simulink model "OpenSeesPy_Simulink"  (R2021a)
settings: Solver=ode8  StartTime=0.0  StopTime=31.2  FixedStep=dtfast  RelTol=1e-3
PreLoadFcn:
  | initializeSimulation;
InitFcn:
  | clear('all');
  | initializeSimulation;
undefined symbols (not defined in the file): adaptive, Area, areaC, asiv, Be, Cl, coef, damperA, damperB, damperC, damperCanon, denfilter, DiscIntNeverNeededParam, dtsim, f, fir_coef, flowCanon, forceCanon, forgfact, frictionA, frictionB, frictionC, gasConstant, Gsnsr_DT, Gsnsr_FT, Kc, ke, kgap, khard, Kp, Kq, kv, learningrate, lengthCanon, massA, massB, massC, massCanon, maxDisplA, maxDisplB, maxDisplC, maxForceC, maxOilVolume, maxVelocA, maxVelocB, maxVelocC, minDisplA, minDisplB, minDisplC, minVelocA, minVelocB, minVelocC, n1siv, n2siv, Ngap, nsiv, numfilter, P_corr_i, precharge, pumpFlow ... (+25)
libraries: simulink x4, instrumentlib x2, dsparch4 x1, sldrtlib x1
(part 2 of 3)

== system OpenSeesPy_Simulink/MTS actuator/static channel #3/payload ==
  force : Inport
  Sum : Sum  Inputs=+----  InputSameDT=on  SaturateOnIntegerOverflow=on  OutDataTypeStr=Inherit: Same as first input
  damper : Gain  Gain=damperC*damperCanon  SaturateOnIntegerOverflow=on  OutDataTypeStr=Inherit: Same as input  ParamDataTypeStr=Inherit: Same as input
  div : Product  Inputs=*/  InputSameDT=on  SaturateOnIntegerOverflow=on  OutDataTypeStr=Inherit: Same as first input
  double integrator : Subsystem
  friction : Subsystem  mask{friction=frictionC*forceCanon, yieldDispl=yieldDisplC*lengthCanon, hysteresis=0}
      mask prompts: friction "Sliding friction"; yieldDispl "Equiv. yield displacement (in)"; hysteresis "Hysteresis constant"
  mass : Constant  Value=massC*massCanon
  static force : Constant  Value=staticForceC*forceCanon
  term1 : Terminator
  unit dly : UnitDelay  SampleTime=-1  HasFrameUpgradeWarning=on
  unit dly1 : UnitDelay  SampleTime=-1  HasFrameUpgradeWarning=on
  veloc units : Gain  Gain=1/velocCanon  SaturateOnIntegerOverflow=on  OutDataTypeStr=Inherit: Same as input  ParamDataTypeStr=Inherit: Same as input
  displ : Outport
  veloc : Outport  Port=2
  tag scope: ch7a=global
  wires:
  unit dly/1 -> [ch7a]
  [ch7b] -> Sum/3  "spring force"
  unit dly1/1 -> damper/1
  damper/1 -> Sum/4  "damper force"
  static force/1 -> Sum/5  "static force"
  double integrator/2(veloc) -> unit dly1/1, friction/1(veloc), veloc units/1
  double integrator/1(displ) -> unit dly/1, displ/1
  div/1 -> double integrator/1(accel)
  double integrator/3(acc) -> term1/1
  mass/1 -> div/2
  force/1 -> Sum/1  "total force"
  Sum/1 -> div/1  "inertial force"
  veloc units/1 -> veloc/1
  friction/1(force) -> Sum/2  "friction force"

== system OpenSeesPy_Simulink/MTS actuator/static channel #4/actuator//valve model ==
  note: Parameter vector:
      | 1:   oil bulk modulus (force/displ^2)
      | 2:   servovalve delay (sec)
      | 3:   servovalve overlap
      | 4:   rated pressure (force/displ^2)
      | 5:   rated flow at rated pressure (displ^3/sec)
      | 6:   nominal flow at rated pressure (displ^3/sec)
      | 7:   actuator piston area 1 (displ^2)
      | 8:   actuator piston area 2 (displ^2)
      | 9:   actuator usable stroke 1 (displ)
      | 10: actuator usable stroke 2 (displ)
      | 11: actuator end cushion length 1 (displ)
      | 12: actuator end cushion length 2 (displ)
      | 13: actuator parasitic damping factor
      | 14: cross-chamber leakage factor (flow/press)
      | 15: ratio port openings according to area
      | 16: sample period (sec)
      |
      | Conversion factors used for converting
      | signals from external (user) to internal
      | (canonical) units:
      |
      | 17: displacement
      | 18: velocity
      | 19: force
      | 20: pressure
      | 21: flow
  note: Note: "1" and "2" denote actuator
      | cylinders on either side of the
      | actuator piston.  With positive
      | valve drive, oil is ported into
      | cylinder 1, resulting in positive
      | displacement.
  note: Auxiliary diagnostic output vector:
      | 1:   valve opening
      | 2:   C1 pressure
      | 3:   C2 pressure
      | 4:   delta pressure
      | 5:   force
      | 6:   velocity
      | 7:   C1 flow
      | 8:   C2 flow
      | 9:   total flow
      | 10: kinematic flow
      | 11: compressibility flow
      | 12: leakage flow
  cmd : Inport
  displ : Inport  Port=2
  veloc : Inport  Port=3
  spl press : Inport  Port=4
  rtn press : Inport  Port=5
  abs : Abs  SaturateOnIntegerOverflow=on
  actuator : S-Function  FunctionName=actuator  Parameters=actParamsC  SFunctionDeploymentMode=off  EnableBusSupport=off
  total flow sel : Selector  InputPortWidth=12  IndexOptions=Index vector (dialog)  Indices=9  OutputSizes=1
  force : Outport
  flow : Outport  Port=2
  wires:
  veloc/1 -> actuator/3
  displ/1 -> actuator/2
  actuator/1 -> force/1
  cmd/1 -> actuator/1
  rtn press/1 -> actuator/5
  spl press/1 -> actuator/4
  total flow sel/1 -> abs/1
  actuator/2 -> total flow sel/1
  abs/1 -> flow/1

== system OpenSeesPy_Simulink/MTS actuator/static channel #4/payload ==
  force : Inport
  Sum : Sum  Inputs=+----  InputSameDT=on  SaturateOnIntegerOverflow=on  OutDataTypeStr=Inherit: Same as first input
  damper : Gain  Gain=damperC*damperCanon  SaturateOnIntegerOverflow=on  OutDataTypeStr=Inherit: Same as input  ParamDataTypeStr=Inherit: Same as input
  div : Product  Inputs=*/  InputSameDT=on  SaturateOnIntegerOverflow=on  OutDataTypeStr=Inherit: Same as first input
  double integrator : Subsystem
  friction : Subsystem  mask{friction=frictionC*forceCanon, yieldDispl=yieldDisplC*lengthCanon, hysteresis=0}
      mask prompts: friction "Sliding friction"; yieldDispl "Equiv. yield displacement (in)"; hysteresis "Hysteresis constant"
  mass : Constant  Value=massC*massCanon
  static force : Constant  Value=staticForceC*forceCanon
  term1 : Terminator
  unit dly : UnitDelay  SampleTime=-1  HasFrameUpgradeWarning=on
  unit dly1 : UnitDelay  SampleTime=-1  HasFrameUpgradeWarning=on
  veloc units : Gain  Gain=1/velocCanon  SaturateOnIntegerOverflow=on  OutDataTypeStr=Inherit: Same as input  ParamDataTypeStr=Inherit: Same as input
  displ : Outport
  veloc : Outport  Port=2
  tag scope: ch8a=global
  wires:
  unit dly/1 -> [ch8a]
  [ch8b] -> Sum/3  "spring force"
  unit dly1/1 -> damper/1
  damper/1 -> Sum/4  "damper force"
  static force/1 -> Sum/5  "static force"
  double integrator/2(veloc) -> unit dly1/1, friction/1(veloc), veloc units/1
  double integrator/1(displ) -> unit dly/1, displ/1
  div/1 -> double integrator/1(accel)
  double integrator/3(acc) -> term1/1
  mass/1 -> div/2
  force/1 -> Sum/1  "total force"
  Sum/1 -> div/1  "inertial force"
  veloc units/1 -> veloc/1
  friction/1(force) -> Sum/2  "friction force"

== system OpenSeesPy_Simulink/Plant/Subsystem/Hardening-spring ==
  x : Inport
  Constant1 : Constant  Value=khard
  MATLAB Function : MATLAB Function  TreatAsAtomicUnit=on
  To Workspace : ToWorkspace  VariableName=Fhard  SaveFormat=Timeseries  SampleTime=-1
  Unit Delay : UnitDelay  SampleTime=-1  HasFrameUpgradeWarning=on
  Fhard : Outport  VectorParamsAs1DForOutWhenUnconnected=off
  wires:
  x/1 -> Unit Delay/1
  Constant1/1 -> MATLAB Function/2(khard)
  MATLAB Function/1(Fhard) -> Fhard/1, To Workspace/1
  Unit Delay/1 -> MATLAB Function/1(x)

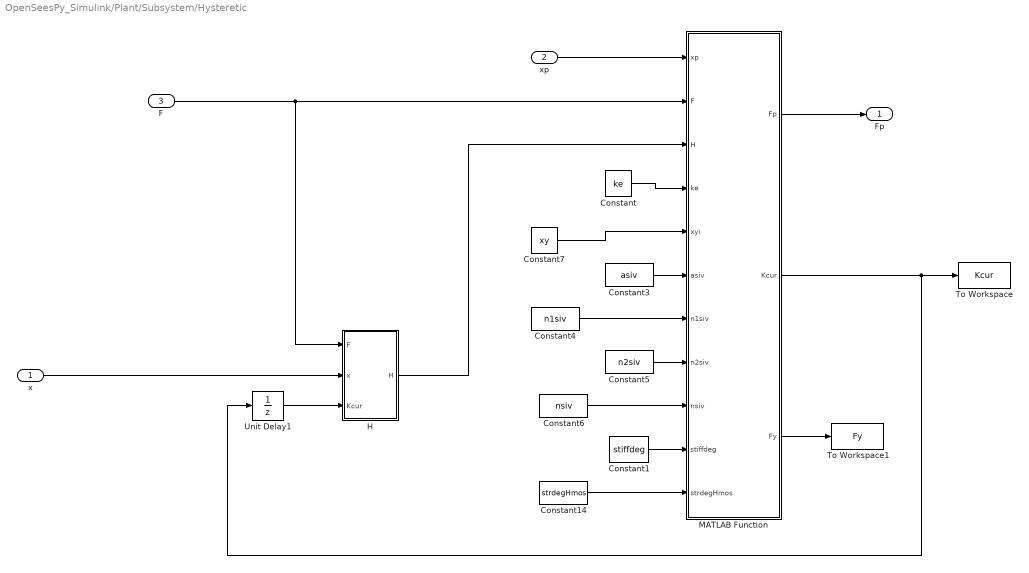
== system OpenSeesPy_Simulink/Plant/Subsystem/Hysteretic ==
  x : Inport
  xp : Inport  Port=2
  F : Inport  Port=3
  Constant : Constant  Value=ke
  Constant1 : Constant  Value=stiffdeg
  Constant14 : Constant  Value=strdegHmos
  Constant3 : Constant  Value=asiv
  Constant4 : Constant  Value=n1siv
  Constant5 : Constant  Value=n2siv
  Constant6 : Constant  Value=nsiv
  Constant7 : Constant  Value=xy
  H : Subsystem
  MATLAB Function : MATLAB Function  TreatAsAtomicUnit=on
  To Workspace : ToWorkspace  VariableName=Kcur  SaveFormat=Timeseries  SampleTime=-1
  To Workspace1 : ToWorkspace  VariableName=Fy  SaveFormat=Timeseries  SampleTime=-1
  Unit Delay1 : UnitDelay  InitialCondition=ke  SampleTime=-1  HasFrameUpgradeWarning=on
  Fp : Outport  VectorParamsAs1DForOutWhenUnconnected=off
  wires:
  MATLAB Function/1(Fp) -> Fp/1
  MATLAB Function/2(Kcur) -> To Workspace/1, Unit Delay1/1
  x/1 -> H/2(x)
  xp/1 -> MATLAB Function/1(xp)
  Constant/1 -> MATLAB Function/4(ke)
  Constant7/1 -> MATLAB Function/5(xyi)
  Constant1/1 -> MATLAB Function/10(stiffdeg)
  Constant3/1 -> MATLAB Function/6(asiv)
  Constant4/1 -> MATLAB Function/7(n1siv)
  Constant5/1 -> MATLAB Function/8(n2siv)
  Constant6/1 -> MATLAB Function/9(nsiv)
  H/1(H) -> MATLAB Function/3(H)
  Unit Delay1/1 -> H/3("Kcur ")
  F/1 -> MATLAB Function/2(F), H/1(F)
  MATLAB Function/3(Fy) -> To Workspace1/1
  Constant14/1 -> MATLAB Function/11(strdegHmos)

== system OpenSeesPy_Simulink/Plant/Subsystem/gapclosing ==
  x : Inport
  Constant : Constant  Value=ke
  Constant1 : Constant  Value=kgap
  Constant7 : Constant  Value=Ngap
  Constant8 : Constant  Value=xgap
  MATLAB Function : MATLAB Function  TreatAsAtomicUnit=on
  To Workspace : ToWorkspace  VariableName=Fgap  SaveFormat=Timeseries  SampleTime=-1
  Unit Delay : UnitDelay  SampleTime=-1  HasFrameUpgradeWarning=on
  Fgap : Outport  VectorParamsAs1DForOutWhenUnconnected=off
  wires:
  Constant7/1 -> MATLAB Function/4(Ngap)
  MATLAB Function/1(Fgap) -> To Workspace/1, Fgap/1
  Constant1/1 -> MATLAB Function/2(kgap)
  Constant8/1 -> MATLAB Function/5(xgap)
  Constant/1 -> MATLAB Function/3(ke)
  x/1 -> Unit Delay/1
  Unit Delay/1 -> MATLAB Function/1(x)

== system OpenSeesPy_Simulink/Wiener Implementation/Prediction_Adaptive_Fixed/Contador ==
  Add : Sum
  Constant1 : Constant
  Unit Delay : UnitDelay  SampleTime=-1  HasFrameUpgradeWarning=on
  Out1 : Outport
  wires:
  Unit Delay/1 -> Add/2
  Constant1/1 -> Add/1
  Add/1 -> Out1/1, Unit Delay/1

== system OpenSeesPy_Simulink/Wiener Implementation/Prediction_Adaptive_Fixed/If Action Subsystem ==
  Disp : Inport
  lambda : Inport  Port=2
  Disp_Pred : Inport  Port=3
  Action Port : ActionPort  ActionPortLabel=if(u1 <2)
  Add : Sum
  Buffer1 : Buffer  N=8  V=7  OutputFrames=off
  Constant1 : Constant
  Constant2 : Constant  Value=w_80
  Gain : Gain  Gain=1e-10
  Product : Product
  Product1 : Product  Inputs=3
  Sum : Sum  Inputs=|+-
  Sum1 : Sum  Inputs=|+-
  Unit Delay : UnitDelay  SampleTime=-1  HasFrameUpgradeWarning=on
  W_new : Outport
  wires:
  lambda/1 -> Product1/1, Gain/1
  Gain/1 -> Sum1/2
  Add/1 -> W_new/1
  Constant2/1 -> Product/1
  Buffer1/1 -> Product1/2
  Product1/1 -> Add/2
  Product/1 -> Add/1
  Disp/1 -> Buffer1/1, Sum/1
  Sum1/1 -> Product/2
  Sum/1 -> Product1/3
  Unit Delay/1 -> Sum/2
  Constant1/1 -> Sum1/1
  Disp_Pred/1 -> Unit Delay/1

== system OpenSeesPy_Simulink/Wiener Implementation/Prediction_Adaptive_Fixed/If Action Subsystem1 ==
  Disp : Inport
  W_prev : Inport  Port=2
  lambda : Inport  Port=3
  Disp_Pred : Inport  Port=4
  Action Port : ActionPort  ActionPortLabel=else
  Add : Sum
  Buffer1 : Buffer  N=8  V=7  OutputFrames=off
  Constant1 : Constant
  Gain : Gain  Gain=1e-10
  Product : Product
  Product1 : Product  Inputs=3
  Sum : Sum  Inputs=|+-
  Sum1 : Sum  Inputs=|+-
  Unit Delay : UnitDelay  SampleTime=-1  HasFrameUpgradeWarning=on
  W_new : Outport
  wires:
  lambda/1 -> Product1/1, Gain/1
  Gain/1 -> Sum1/2
  Add/1 -> W_new/1
  W_prev/1 -> Product/1
  Buffer1/1 -> Product1/2
  Product1/1 -> Add/2
  Product/1 -> Add/1
  Disp/1 -> Buffer1/1, Sum/1
  Sum1/1 -> Product/2
  Sum/1 -> Product1/3
  Unit Delay/1 -> Sum/2
  Constant1/1 -> Sum1/1
  Disp_Pred/1 -> Unit Delay/1

== system OpenSeesPy_Simulink/Wiener Implementation/Test3/Subsystem ==
  Constant1 : Constant
  Constant3 : Constant  Value=2
  Constant5 : Constant  Value=3
  Constant6 : Constant  Value=0
  Constant7 : Constant  Value=x02
  Math Function{,1..3} (4 alike) : Math  Operator=pow  SaturateOnIntegerOverflow=on
  Matrix Concatenate : Concatenate  NumInputs=4  Mode=Multidimensional array  ConcatenateDimension=2
  a : Outport
  wires:
  Constant6/1 -> Math Function/2
  Constant1/1 -> Math Function1/2
  Constant3/1 -> Math Function2/2
  Constant5/1 -> Math Function3/2
  Math Function/1 -> Matrix Concatenate/1
  Math Function1/1 -> Matrix Concatenate/2
  Math Function2/1 -> Matrix Concatenate/3
  Math Function3/1 -> Matrix Concatenate/4
  Matrix Concatenate/1 -> a/1  "a"
  Constant7/1 -> Math Function3/1, Math Function2/1, Math Function1/1, Math Function/1

== system OpenSeesPy_Simulink/MTS actuator/dynamic long channel #1/payload/double integrator ==
  accel : Inport
  displ gen : DiscreteIntegrator  IntegratorMethod=Integration: Backward Euler  SampleTime=1/4000  LimitOutput=on  UpperSaturationLimit=maxDisplB*coef  LowerSaturationLimit=minDisplB*coef  ShowSaturationPort=on  ICPrevOutput=DiscIntNeverNeededParam  ICPrevScaledInput=DiscIntNeverNeededParam
  veloc gen : Subsystem  mask{maxVeloc=maxVelocB*velocCanon*coef, minVeloc=minVelocB*velocCanon*coef, maxDispl=maxDisplB*coef, minDispl=minDisplB*coef}
      mask prompts: maxVeloc "Max velocity"; minVeloc "Min velocity"; maxDispl "Max displacement"; minDispl "Min displacement"
  displ : Outport
  veloc : Outport  Port=2
  acc : Outport  Port=3
  wires:
  accel/1 -> acc/1, veloc gen/1(accel)
  veloc gen/1(veloc) -> veloc/1, displ gen/1
  displ gen/1 -> veloc gen/2(displ), displ/1
  displ gen/2 -> veloc gen/3(reset)

== system OpenSeesPy_Simulink/MTS actuator/dynamic long channel #1/payload/friction ==
  veloc : Inport
  1-beta : Gain  Gain=1-hysteresis  SaturateOnIntegerOverflow=on  OutDataTypeStr=Inherit: Same as input  ParamDataTypeStr=Inherit: Same as input
  Sign : Signum
  Sum : Sum  Inputs=|++  SaturateOnIntegerOverflow=on
  Sum1 : Sum  Inputs=|+-  SaturateOnIntegerOverflow=on
  beta : Constant  Value=hysteresis
  integrator : DiscreteIntegrator  SampleTime=-1  LimitOutput=on  UpperSaturationLimit=1  LowerSaturationLimit=-1  ICPrevOutput=DiscIntNeverNeededParam  ICPrevScaledInput=DiscIntNeverNeededParam
  one : Constant
  prod1 : Product  InputSameDT=on  SaturateOnIntegerOverflow=on  OutDataTypeStr=Inherit: Same as first input
  prod2 : Product  InputSameDT=on  SaturateOnIntegerOverflow=on  OutDataTypeStr=Inherit: Same as first input
  prod3 : Product  Inputs=3  InputSameDT=on  SaturateOnIntegerOverflow=on  OutDataTypeStr=Inherit: Same as first input
  prod4 : Product  InputSameDT=on  SaturateOnIntegerOverflow=on  OutDataTypeStr=Inherit: Same as first input
  sliding friction : Constant  Value=friction
  y inv : Gain  Gain=1/max(eps, yieldDispl)  SaturateOnIntegerOverflow=on  OutDataTypeStr=Inherit: Same as input  ParamDataTypeStr=Inherit: Same as input
  force : Outport
  wires:
  integrator/1 -> prod3/2, prod3/1, prod4/1, prod1/2  "zee"
  y inv/1 -> integrator/1
  prod2/1 -> y inv/1
  Sum1/1 -> prod2/1
  prod3/1 -> Sum1/2
  one/1 -> Sum1/1
  Sum/1 -> prod3/3
  beta/1 -> Sum/1
  1-beta/1 -> Sum/2
  Sign/1 -> 1-beta/1
  prod4/1 -> Sign/1
  veloc/1 -> prod2/2, prod4/2
  prod1/1 -> force/1
  sliding friction/1 -> prod1/1

== system OpenSeesPy_Simulink/MTS actuator/dynamic long channel #2/payload/double integrator ==
  accel : Inport
  displ gen : DiscreteIntegrator  IntegratorMethod=Integration: Backward Euler  SampleTime=-1  LimitOutput=on  UpperSaturationLimit=maxDisplB  LowerSaturationLimit=minDisplB  ShowSaturationPort=on  ICPrevOutput=DiscIntNeverNeededParam  ICPrevScaledInput=DiscIntNeverNeededParam
  veloc gen : Subsystem  mask{maxVeloc=maxVelocB*velocCanon, minVeloc=minVelocB*velocCanon, maxDispl=maxDisplB, minDispl=minDisplB}
      mask prompts: maxVeloc "Max velocity"; minVeloc "Min velocity"; maxDispl "Max displacement"; minDispl "Min displacement"
  displ : Outport
  veloc : Outport  Port=2
  acc : Outport  Port=3
  wires:
  accel/1 -> acc/1, veloc gen/1(accel)
  veloc gen/1(veloc) -> veloc/1, displ gen/1
  displ gen/1 -> veloc gen/2(displ), displ/1
  displ gen/2 -> veloc gen/3(reset)

== system OpenSeesPy_Simulink/MTS actuator/dynamic long channel #2/payload/friction ==
  veloc : Inport
  1-beta : Gain  Gain=1-hysteresis  SaturateOnIntegerOverflow=on  OutDataTypeStr=Inherit: Same as input  ParamDataTypeStr=Inherit: Same as input
  Sign : Signum
  Sum : Sum  Inputs=|++  SaturateOnIntegerOverflow=on
  Sum1 : Sum  Inputs=|+-  SaturateOnIntegerOverflow=on
  beta : Constant  Value=hysteresis
  integrator : DiscreteIntegrator  SampleTime=-1  LimitOutput=on  UpperSaturationLimit=1  LowerSaturationLimit=-1  ICPrevOutput=DiscIntNeverNeededParam  ICPrevScaledInput=DiscIntNeverNeededParam
  one : Constant
  prod1 : Product  InputSameDT=on  SaturateOnIntegerOverflow=on  OutDataTypeStr=Inherit: Same as first input
  prod2 : Product  InputSameDT=on  SaturateOnIntegerOverflow=on  OutDataTypeStr=Inherit: Same as first input
  prod3 : Product  Inputs=3  InputSameDT=on  SaturateOnIntegerOverflow=on  OutDataTypeStr=Inherit: Same as first input
  prod4 : Product  InputSameDT=on  SaturateOnIntegerOverflow=on  OutDataTypeStr=Inherit: Same as first input
  sliding friction : Constant  Value=friction
  y inv : Gain  Gain=1/max(eps, yieldDispl)  SaturateOnIntegerOverflow=on  OutDataTypeStr=Inherit: Same as input  ParamDataTypeStr=Inherit: Same as input
  force : Outport
  wires:
  integrator/1 -> prod3/2, prod3/1, prod4/1, prod1/2  "zee"
  y inv/1 -> integrator/1
  prod2/1 -> y inv/1
  Sum1/1 -> prod2/1
  prod3/1 -> Sum1/2
  one/1 -> Sum1/1
  Sum/1 -> prod3/3
  beta/1 -> Sum/1
  1-beta/1 -> Sum/2
  Sign/1 -> 1-beta/1
  prod4/1 -> Sign/1
  veloc/1 -> prod2/2, prod4/2
  prod1/1 -> force/1
  sliding friction/1 -> prod1/1

== system OpenSeesPy_Simulink/MTS actuator/dynamic short channel #1/payload/double integrator ==
  accel : Inport
  displ gen : DiscreteIntegrator  IntegratorMethod=Integration: Backward Euler  SampleTime=1/1024  LimitOutput=on  UpperSaturationLimit=maxDisplA  LowerSaturationLimit=minDisplA  ShowSaturationPort=on  ICPrevOutput=DiscIntNeverNeededParam  ICPrevScaledInput=DiscIntNeverNeededParam
  veloc gen : Subsystem  mask{maxVeloc=maxVelocA*velocCanon, minVeloc=minVelocA*velocCanon, maxDispl=maxDisplA, minDispl=minDisplA}
      mask prompts: maxVeloc "Max velocity"; minVeloc "Min velocity"; maxDispl "Max displacement"; minDispl "Min displacement"
  displ : Outport
  veloc : Outport  Port=2
  acc : Outport  Port=3
  wires:
  accel/1 -> acc/1, veloc gen/1(accel)
  veloc gen/1(veloc) -> veloc/1, displ gen/1
  displ gen/1 -> veloc gen/2(displ), displ/1
  displ gen/2 -> veloc gen/3(reset)

== system OpenSeesPy_Simulink/MTS actuator/dynamic short channel #1/payload/friction ==
  veloc : Inport
  1-beta : Gain  Gain=1-hysteresis  SaturateOnIntegerOverflow=on  OutDataTypeStr=Inherit: Same as input  ParamDataTypeStr=Inherit: Same as input
  Sign : Signum
  Sum : Sum  Inputs=|++  SaturateOnIntegerOverflow=on
  Sum1 : Sum  Inputs=|+-  SaturateOnIntegerOverflow=on
  beta : Constant  Value=hysteresis
  integrator : DiscreteIntegrator  SampleTime=-1  LimitOutput=on  UpperSaturationLimit=1  LowerSaturationLimit=-1  ICPrevOutput=DiscIntNeverNeededParam  ICPrevScaledInput=DiscIntNeverNeededParam
  one : Constant
  prod1 : Product  InputSameDT=on  SaturateOnIntegerOverflow=on  OutDataTypeStr=Inherit: Same as first input
  prod2 : Product  InputSameDT=on  SaturateOnIntegerOverflow=on  OutDataTypeStr=Inherit: Same as first input
  prod3 : Product  Inputs=3  InputSameDT=on  SaturateOnIntegerOverflow=on  OutDataTypeStr=Inherit: Same as first input
  prod4 : Product  InputSameDT=on  SaturateOnIntegerOverflow=on  OutDataTypeStr=Inherit: Same as first input
  sliding friction : Constant  Value=friction
  y inv : Gain  Gain=1/max(eps, yieldDispl)  SaturateOnIntegerOverflow=on  OutDataTypeStr=Inherit: Same as input  ParamDataTypeStr=Inherit: Same as input
  force : Outport
  wires:
  integrator/1 -> prod3/2, prod3/1, prod4/1, prod1/2  "zee"
  y inv/1 -> integrator/1
  prod2/1 -> y inv/1
  Sum1/1 -> prod2/1
  prod3/1 -> Sum1/2
  one/1 -> Sum1/1
  Sum/1 -> prod3/3
  beta/1 -> Sum/1
  1-beta/1 -> Sum/2
  Sign/1 -> 1-beta/1
  prod4/1 -> Sign/1
  veloc/1 -> prod2/2, prod4/2
  prod1/1 -> force/1
  sliding friction/1 -> prod1/1

== system OpenSeesPy_Simulink/MTS actuator/dynamic short channel #2/payload/double integrator ==
  accel : Inport
  displ gen : DiscreteIntegrator  IntegratorMethod=Integration: Backward Euler  SampleTime=-1  LimitOutput=on  UpperSaturationLimit=maxDisplA  LowerSaturationLimit=minDisplA  ShowSaturationPort=on  ICPrevOutput=DiscIntNeverNeededParam  ICPrevScaledInput=DiscIntNeverNeededParam
  veloc gen : Subsystem  mask{maxVeloc=maxVelocA*velocCanon, minVeloc=minVelocA*velocCanon, maxDispl=maxDisplA, minDispl=minDisplA}
      mask prompts: maxVeloc "Max velocity"; minVeloc "Min velocity"; maxDispl "Max displacement"; minDispl "Min displacement"
  displ : Outport
  veloc : Outport  Port=2
  acc : Outport  Port=3
  wires:
  accel/1 -> acc/1, veloc gen/1(accel)
  veloc gen/1(veloc) -> veloc/1, displ gen/1
  displ gen/1 -> veloc gen/2(displ), displ/1
  displ gen/2 -> veloc gen/3(reset)

== system OpenSeesPy_Simulink/MTS actuator/dynamic short channel #2/payload/friction ==
  veloc : Inport
  1-beta : Gain  Gain=1-hysteresis  SaturateOnIntegerOverflow=on  OutDataTypeStr=Inherit: Same as input  ParamDataTypeStr=Inherit: Same as input
  Sign : Signum
  Sum : Sum  Inputs=|++  SaturateOnIntegerOverflow=on
  Sum1 : Sum  Inputs=|+-  SaturateOnIntegerOverflow=on
  beta : Constant  Value=hysteresis
  integrator : DiscreteIntegrator  SampleTime=-1  LimitOutput=on  UpperSaturationLimit=1  LowerSaturationLimit=-1  ICPrevOutput=DiscIntNeverNeededParam  ICPrevScaledInput=DiscIntNeverNeededParam
  one : Constant
  prod1 : Product  InputSameDT=on  SaturateOnIntegerOverflow=on  OutDataTypeStr=Inherit: Same as first input
  prod2 : Product  InputSameDT=on  SaturateOnIntegerOverflow=on  OutDataTypeStr=Inherit: Same as first input
  prod3 : Product  Inputs=3  InputSameDT=on  SaturateOnIntegerOverflow=on  OutDataTypeStr=Inherit: Same as first input
  prod4 : Product  InputSameDT=on  SaturateOnIntegerOverflow=on  OutDataTypeStr=Inherit: Same as first input
  sliding friction : Constant  Value=friction
  y inv : Gain  Gain=1/max(eps, yieldDispl)  SaturateOnIntegerOverflow=on  OutDataTypeStr=Inherit: Same as input  ParamDataTypeStr=Inherit: Same as input
  force : Outport
  wires:
  integrator/1 -> prod3/2, prod3/1, prod4/1, prod1/2  "zee"
  y inv/1 -> integrator/1
  prod2/1 -> y inv/1
  Sum1/1 -> prod2/1
  prod3/1 -> Sum1/2
  one/1 -> Sum1/1
  Sum/1 -> prod3/3
  beta/1 -> Sum/1
  1-beta/1 -> Sum/2
  Sign/1 -> 1-beta/1
  prod4/1 -> Sign/1
  veloc/1 -> prod2/2, prod4/2
  prod1/1 -> force/1
  sliding friction/1 -> prod1/1

== system OpenSeesPy_Simulink/MTS actuator/static channel #1/payload/double integrator ==
  accel : Inport
  displ gen : DiscreteIntegrator  IntegratorMethod=Integration: Backward Euler  SampleTime=-1  LimitOutput=on  UpperSaturationLimit=maxDisplC  LowerSaturationLimit=minDisplC  ShowSaturationPort=on  ICPrevOutput=DiscIntNeverNeededParam  ICPrevScaledInput=DiscIntNeverNeededParam
  veloc gen : Subsystem  mask{maxVeloc=maxVelocC*velocCanon, minVeloc=minVelocC*velocCanon, maxDispl=maxDisplC, minDispl=minDisplC}
      mask prompts: maxVeloc "Max velocity"; minVeloc "Min velocity"; maxDispl "Max displacement"; minDispl "Min displacement"
  displ : Outport
  veloc : Outport  Port=2
  acc : Outport  Port=3
  wires:
  accel/1 -> acc/1, veloc gen/1(accel)
  veloc gen/1(veloc) -> veloc/1, displ gen/1
  displ gen/1 -> veloc gen/2(displ), displ/1
  displ gen/2 -> veloc gen/3(reset)

== system OpenSeesPy_Simulink/MTS actuator/static channel #1/payload/friction ==
  veloc : Inport
  1-beta : Gain  Gain=1-hysteresis  SaturateOnIntegerOverflow=on  OutDataTypeStr=Inherit: Same as input  ParamDataTypeStr=Inherit: Same as input
  Sign : Signum
  Sum : Sum  Inputs=|++  SaturateOnIntegerOverflow=on
  Sum1 : Sum  Inputs=|+-  SaturateOnIntegerOverflow=on
  beta : Constant  Value=hysteresis
  integrator : DiscreteIntegrator  SampleTime=-1  LimitOutput=on  UpperSaturationLimit=1  LowerSaturationLimit=-1  ICPrevOutput=DiscIntNeverNeededParam  ICPrevScaledInput=DiscIntNeverNeededParam
  one : Constant
  prod1 : Product  InputSameDT=on  SaturateOnIntegerOverflow=on  OutDataTypeStr=Inherit: Same as first input
  prod2 : Product  InputSameDT=on  SaturateOnIntegerOverflow=on  OutDataTypeStr=Inherit: Same as first input
  prod3 : Product  Inputs=3  InputSameDT=on  SaturateOnIntegerOverflow=on  OutDataTypeStr=Inherit: Same as first input
  prod4 : Product  InputSameDT=on  SaturateOnIntegerOverflow=on  OutDataTypeStr=Inherit: Same as first input
  sliding friction : Constant  Value=friction
  y inv : Gain  Gain=1/max(eps, yieldDispl)  SaturateOnIntegerOverflow=on  OutDataTypeStr=Inherit: Same as input  ParamDataTypeStr=Inherit: Same as input
  force : Outport
  wires:
  integrator/1 -> prod3/2, prod3/1, prod4/1, prod1/2  "zee"
  y inv/1 -> integrator/1
  prod2/1 -> y inv/1
  Sum1/1 -> prod2/1
  prod3/1 -> Sum1/2
  one/1 -> Sum1/1
  Sum/1 -> prod3/3
  beta/1 -> Sum/1
  1-beta/1 -> Sum/2
  Sign/1 -> 1-beta/1
  prod4/1 -> Sign/1
  veloc/1 -> prod2/2, prod4/2
  prod1/1 -> force/1
  sliding friction/1 -> prod1/1

== system OpenSeesPy_Simulink/MTS actuator/static channel #2/payload/double integrator ==
  accel : Inport
  displ gen : DiscreteIntegrator  IntegratorMethod=Integration: Backward Euler  SampleTime=-1  LimitOutput=on  UpperSaturationLimit=maxDisplC  LowerSaturationLimit=minDisplC  ShowSaturationPort=on  ICPrevOutput=DiscIntNeverNeededParam  ICPrevScaledInput=DiscIntNeverNeededParam
  veloc gen : Subsystem  mask{maxVeloc=maxVelocC*velocCanon, minVeloc=minVelocC*velocCanon, maxDispl=maxDisplC, minDispl=minDisplC}
      mask prompts: maxVeloc "Max velocity"; minVeloc "Min velocity"; maxDispl "Max displacement"; minDispl "Min displacement"
  displ : Outport
  veloc : Outport  Port=2
  acc : Outport  Port=3
  wires:
  accel/1 -> acc/1, veloc gen/1(accel)
  veloc gen/1(veloc) -> veloc/1, displ gen/1
  displ gen/1 -> veloc gen/2(displ), displ/1
  displ gen/2 -> veloc gen/3(reset)

== system OpenSeesPy_Simulink/MTS actuator/static channel #2/payload/friction ==
  veloc : Inport
  1-beta : Gain  Gain=1-hysteresis  SaturateOnIntegerOverflow=on  OutDataTypeStr=Inherit: Same as input  ParamDataTypeStr=Inherit: Same as input
  Sign : Signum
  Sum : Sum  Inputs=|++  SaturateOnIntegerOverflow=on
  Sum1 : Sum  Inputs=|+-  SaturateOnIntegerOverflow=on
  beta : Constant  Value=hysteresis
  integrator : DiscreteIntegrator  SampleTime=-1  LimitOutput=on  UpperSaturationLimit=1  LowerSaturationLimit=-1  ICPrevOutput=DiscIntNeverNeededParam  ICPrevScaledInput=DiscIntNeverNeededParam
  one : Constant
  prod1 : Product  InputSameDT=on  SaturateOnIntegerOverflow=on  OutDataTypeStr=Inherit: Same as first input
  prod2 : Product  InputSameDT=on  SaturateOnIntegerOverflow=on  OutDataTypeStr=Inherit: Same as first input
  prod3 : Product  Inputs=3  InputSameDT=on  SaturateOnIntegerOverflow=on  OutDataTypeStr=Inherit: Same as first input
  prod4 : Product  InputSameDT=on  SaturateOnIntegerOverflow=on  OutDataTypeStr=Inherit: Same as first input
  sliding friction : Constant  Value=friction
  y inv : Gain  Gain=1/max(eps, yieldDispl)  SaturateOnIntegerOverflow=on  OutDataTypeStr=Inherit: Same as input  ParamDataTypeStr=Inherit: Same as input
  force : Outport
  wires:
  integrator/1 -> prod3/2, prod3/1, prod4/1, prod1/2  "zee"
  y inv/1 -> integrator/1
  prod2/1 -> y inv/1
  Sum1/1 -> prod2/1
  prod3/1 -> Sum1/2
  one/1 -> Sum1/1
  Sum/1 -> prod3/3
  beta/1 -> Sum/1
  1-beta/1 -> Sum/2
  Sign/1 -> 1-beta/1
  prod4/1 -> Sign/1
  veloc/1 -> prod2/2, prod4/2
  prod1/1 -> force/1
  sliding friction/1 -> prod1/1

== system OpenSeesPy_Simulink/MTS actuator/static channel #3/payload/double integrator ==
  accel : Inport
  displ gen : DiscreteIntegrator  IntegratorMethod=Integration: Backward Euler  SampleTime=-1  LimitOutput=on  UpperSaturationLimit=maxDisplC  LowerSaturationLimit=minDisplC  ShowSaturationPort=on  ICPrevOutput=DiscIntNeverNeededParam  ICPrevScaledInput=DiscIntNeverNeededParam
  veloc gen : Subsystem  mask{maxVeloc=maxVelocC*velocCanon, minVeloc=minVelocC*velocCanon, maxDispl=maxDisplC, minDispl=minDisplC}
      mask prompts: maxVeloc "Max velocity"; minVeloc "Min velocity"; maxDispl "Max displacement"; minDispl "Min displacement"
  displ : Outport
  veloc : Outport  Port=2
  acc : Outport  Port=3
  wires:
  accel/1 -> acc/1, veloc gen/1(accel)
  veloc gen/1(veloc) -> veloc/1, displ gen/1
  displ gen/1 -> veloc gen/2(displ), displ/1
  displ gen/2 -> veloc gen/3(reset)

== system OpenSeesPy_Simulink/MTS actuator/static channel #3/payload/friction ==
  veloc : Inport
  1-beta : Gain  Gain=1-hysteresis  SaturateOnIntegerOverflow=on  OutDataTypeStr=Inherit: Same as input  ParamDataTypeStr=Inherit: Same as input
  Sign : Signum
  Sum : Sum  Inputs=|++  SaturateOnIntegerOverflow=on
  Sum1 : Sum  Inputs=|+-  SaturateOnIntegerOverflow=on
  beta : Constant  Value=hysteresis
  integrator : DiscreteIntegrator  SampleTime=-1  LimitOutput=on  UpperSaturationLimit=1  LowerSaturationLimit=-1  ICPrevOutput=DiscIntNeverNeededParam  ICPrevScaledInput=DiscIntNeverNeededParam
  one : Constant
  prod1 : Product  InputSameDT=on  SaturateOnIntegerOverflow=on  OutDataTypeStr=Inherit: Same as first input
  prod2 : Product  InputSameDT=on  SaturateOnIntegerOverflow=on  OutDataTypeStr=Inherit: Same as first input
  prod3 : Product  Inputs=3  InputSameDT=on  SaturateOnIntegerOverflow=on  OutDataTypeStr=Inherit: Same as first input
  prod4 : Product  InputSameDT=on  SaturateOnIntegerOverflow=on  OutDataTypeStr=Inherit: Same as first input
  sliding friction : Constant  Value=friction
  y inv : Gain  Gain=1/max(eps, yieldDispl)  SaturateOnIntegerOverflow=on  OutDataTypeStr=Inherit: Same as input  ParamDataTypeStr=Inherit: Same as input
  force : Outport
  wires:
  integrator/1 -> prod3/2, prod3/1, prod4/1, prod1/2  "zee"
  y inv/1 -> integrator/1
  prod2/1 -> y inv/1
  Sum1/1 -> prod2/1
  prod3/1 -> Sum1/2
  one/1 -> Sum1/1
  Sum/1 -> prod3/3
  beta/1 -> Sum/1
  1-beta/1 -> Sum/2
  Sign/1 -> 1-beta/1
  prod4/1 -> Sign/1
  veloc/1 -> prod2/2, prod4/2
  prod1/1 -> force/1
  sliding friction/1 -> prod1/1

== system OpenSeesPy_Simulink/MTS actuator/static channel #4/payload/double integrator ==
  accel : Inport
  displ gen : DiscreteIntegrator  IntegratorMethod=Integration: Backward Euler  SampleTime=-1  LimitOutput=on  UpperSaturationLimit=maxDisplC  LowerSaturationLimit=minDisplC  ShowSaturationPort=on  ICPrevOutput=DiscIntNeverNeededParam  ICPrevScaledInput=DiscIntNeverNeededParam
  veloc gen : Subsystem  mask{maxVeloc=maxVelocC*velocCanon, minVeloc=minVelocC*velocCanon, maxDispl=maxDisplC, minDispl=minDisplC}
      mask prompts: maxVeloc "Max velocity"; minVeloc "Min velocity"; maxDispl "Max displacement"; minDispl "Min displacement"
  displ : Outport
  veloc : Outport  Port=2
  acc : Outport  Port=3
  wires:
  accel/1 -> acc/1, veloc gen/1(accel)
  veloc gen/1(veloc) -> veloc/1, displ gen/1
  displ gen/1 -> veloc gen/2(displ), displ/1
  displ gen/2 -> veloc gen/3(reset)

== system OpenSeesPy_Simulink/MTS actuator/static channel #4/payload/friction ==
  veloc : Inport
  1-beta : Gain  Gain=1-hysteresis  SaturateOnIntegerOverflow=on  OutDataTypeStr=Inherit: Same as input  ParamDataTypeStr=Inherit: Same as input
  Sign : Signum
  Sum : Sum  Inputs=|++  SaturateOnIntegerOverflow=on
  Sum1 : Sum  Inputs=|+-  SaturateOnIntegerOverflow=on
  beta : Constant  Value=hysteresis
  integrator : DiscreteIntegrator  SampleTime=-1  LimitOutput=on  UpperSaturationLimit=1  LowerSaturationLimit=-1  ICPrevOutput=DiscIntNeverNeededParam  ICPrevScaledInput=DiscIntNeverNeededParam
  one : Constant
  prod1 : Product  InputSameDT=on  SaturateOnIntegerOverflow=on  OutDataTypeStr=Inherit: Same as first input
  prod2 : Product  InputSameDT=on  SaturateOnIntegerOverflow=on  OutDataTypeStr=Inherit: Same as first input
  prod3 : Product  Inputs=3  InputSameDT=on  SaturateOnIntegerOverflow=on  OutDataTypeStr=Inherit: Same as first input
  prod4 : Product  InputSameDT=on  SaturateOnIntegerOverflow=on  OutDataTypeStr=Inherit: Same as first input
  sliding friction : Constant  Value=friction
  y inv : Gain  Gain=1/max(eps, yieldDispl)  SaturateOnIntegerOverflow=on  OutDataTypeStr=Inherit: Same as input  ParamDataTypeStr=Inherit: Same as input
  force : Outport
  wires:
  integrator/1 -> prod3/2, prod3/1, prod4/1, prod1/2  "zee"
  y inv/1 -> integrator/1
  prod2/1 -> y inv/1
  Sum1/1 -> prod2/1
  prod3/1 -> Sum1/2
  one/1 -> Sum1/1
  Sum/1 -> prod3/3
  beta/1 -> Sum/1
  1-beta/1 -> Sum/2
  Sign/1 -> 1-beta/1
  prod4/1 -> Sign/1
  veloc/1 -> prod2/2, prod4/2
  prod1/1 -> force/1
  sliding friction/1 -> prod1/1

== system OpenSeesPy_Simulink/Plant/Subsystem/Hysteretic/H ==
  F : Inport
  x : Inport  Port=2
  "Kcur " : Inport  Port=3
  Discrete-Time Integrator : DiscreteIntegrator  IntegratorMethod=Accumulation: Trapezoidal  SampleTime=-1  ICPrevOutput=DiscIntNeverNeededParam  ICPrevScaledInput=DiscIntNeverNeededParam
  Fmean : DiscreteFir
  Product : Product  Inputs=*/
  Product1 : Product
  Scope{,1..5} (6 alike) : Scope
  Sum1 : Sum  Inputs=|-+
  dF : DiscreteFir  Coefficients=[1 -1]
  dx : DiscreteFir  Coefficients=[1 -1]
  H : Outport  VectorParamsAs1DForOutWhenUnconnected=off
  wires:
  dF/1 -> Scope1/1, Product/1
  "Kcur "/1 -> Scope2/1, Product/2
  Product1/1 -> Discrete-Time Integrator/1
  Sum1/1 -> Product1/2
  x/1 -> Scope5/1, dx/1
  F/1 -> Fmean/1, dF/1
  Discrete-Time Integrator/1 -> Scope4/1, H/1
  Product/1 -> Sum1/1
  dx/1 -> Scope3/1, Sum1/2
  Fmean/1 -> Scope/1, Product1/1

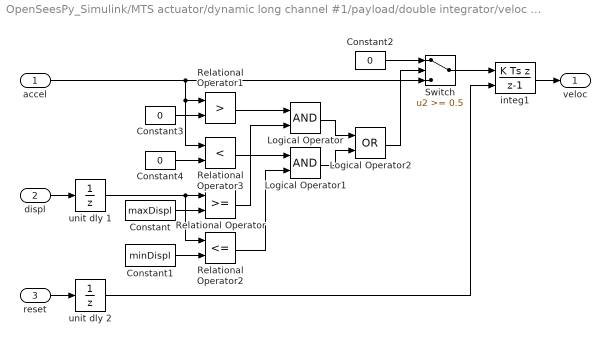
== system OpenSeesPy_Simulink/MTS actuator/dynamic long channel #1/payload/double integrator/veloc gen ==
  accel : Inport
  displ : Inport  Port=2
  reset : Inport  Port=3
  Constant : Constant  Value=maxDispl
  Constant1 : Constant  Value=minDispl
  Constant2 : Constant  Value=0
  Constant3 : Constant  Value=0
  Constant4 : Constant  Value=0
  Logical Operator : Logic
  Logical Operator1 : Logic
  Logical Operator2 : Logic  Operator=OR
  Relational Operator : RelationalOperator  RndMeth=Nearest  InputSameDT=on
  Relational Operator1 : RelationalOperator  Operator=>  RndMeth=Nearest  InputSameDT=on
  Relational Operator2 : RelationalOperator  Operator=<=  RndMeth=Nearest  InputSameDT=on
  Relational Operator3 : RelationalOperator  Operator=<  RndMeth=Nearest  InputSameDT=on
  Switch : Switch  Threshold=0.5  SaturateOnIntegerOverflow=on  InputSameDT=on
  integ1 : DiscreteIntegrator  IntegratorMethod=Integration: Backward Euler  ExternalReset=either  SampleTime=1/4000  LimitOutput=on  UpperSaturationLimit=maxVeloc  LowerSaturationLimit=minVeloc  ICPrevOutput=DiscIntNeverNeededParam  ICPrevScaledInput=DiscIntNeverNeededParam
  unit dly 1 : UnitDelay  SampleTime=-1  HasFrameUpgradeWarning=on
  unit dly 2 : UnitDelay  SampleTime=-1  HasFrameUpgradeWarning=on
  veloc : Outport
  wires:
  integ1/1 -> veloc/1
  Constant/1 -> Relational Operator/2
  Relational Operator/1 -> Logical Operator/2
  Relational Operator2/1 -> Logical Operator1/2
  Constant1/1 -> Relational Operator2/2
  accel/1 -> Relational Operator3/1, Relational Operator1/1, Switch/3
  Constant3/1 -> Relational Operator1/2
  Relational Operator1/1 -> Logical Operator/1
  Constant4/1 -> Relational Operator3/2
  Relational Operator3/1 -> Logical Operator1/1
  Logical Operator/1 -> Logical Operator2/1
  Constant2/1 -> Switch/1
  Logical Operator2/1 -> Switch/2
  Switch/1 -> integ1/1
  unit dly 2/1 -> integ1/2
  Logical Operator1/1 -> Logical Operator2/2
  displ/1 -> unit dly 1/1
  reset/1 -> unit dly 2/1
  unit dly 1/1 -> Relational Operator/1, Relational Operator2/1

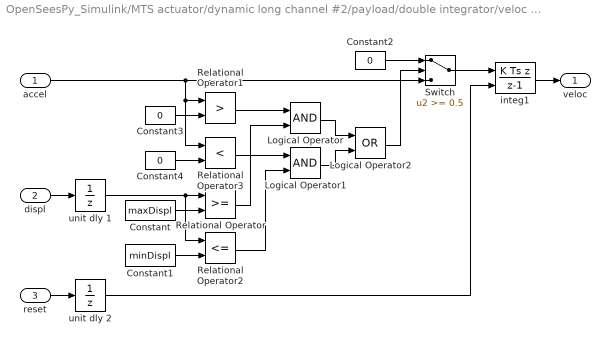
== system OpenSeesPy_Simulink/MTS actuator/dynamic long channel #2/payload/double integrator/veloc gen ==
  accel : Inport
  displ : Inport  Port=2
  reset : Inport  Port=3
  Constant : Constant  Value=maxDispl
  Constant1 : Constant  Value=minDispl
  Constant2 : Constant  Value=0
  Constant3 : Constant  Value=0
  Constant4 : Constant  Value=0
  Logical Operator : Logic
  Logical Operator1 : Logic
  Logical Operator2 : Logic  Operator=OR
  Relational Operator : RelationalOperator  RndMeth=Nearest  InputSameDT=on
  Relational Operator1 : RelationalOperator  Operator=>  RndMeth=Nearest  InputSameDT=on
  Relational Operator2 : RelationalOperator  Operator=<=  RndMeth=Nearest  InputSameDT=on
  Relational Operator3 : RelationalOperator  Operator=<  RndMeth=Nearest  InputSameDT=on
  Switch : Switch  Threshold=0.5  SaturateOnIntegerOverflow=on  InputSameDT=on
  integ1 : DiscreteIntegrator  IntegratorMethod=Integration: Backward Euler  ExternalReset=either  SampleTime=-1  LimitOutput=on  UpperSaturationLimit=maxVeloc  LowerSaturationLimit=minVeloc  ICPrevOutput=DiscIntNeverNeededParam  ICPrevScaledInput=DiscIntNeverNeededParam
  unit dly 1 : UnitDelay  SampleTime=-1  HasFrameUpgradeWarning=on
  unit dly 2 : UnitDelay  SampleTime=-1  HasFrameUpgradeWarning=on
  veloc : Outport
  wires:
  integ1/1 -> veloc/1
  Constant/1 -> Relational Operator/2
  Relational Operator/1 -> Logical Operator/2
  Relational Operator2/1 -> Logical Operator1/2
  Constant1/1 -> Relational Operator2/2
  accel/1 -> Relational Operator3/1, Relational Operator1/1, Switch/3
  Constant3/1 -> Relational Operator1/2
  Relational Operator1/1 -> Logical Operator/1
  Constant4/1 -> Relational Operator3/2
  Relational Operator3/1 -> Logical Operator1/1
  Logical Operator/1 -> Logical Operator2/1
  Constant2/1 -> Switch/1
  Logical Operator2/1 -> Switch/2
  Switch/1 -> integ1/1
  unit dly 2/1 -> integ1/2
  Logical Operator1/1 -> Logical Operator2/2
  displ/1 -> unit dly 1/1
  reset/1 -> unit dly 2/1
  unit dly 1/1 -> Relational Operator/1, Relational Operator2/1

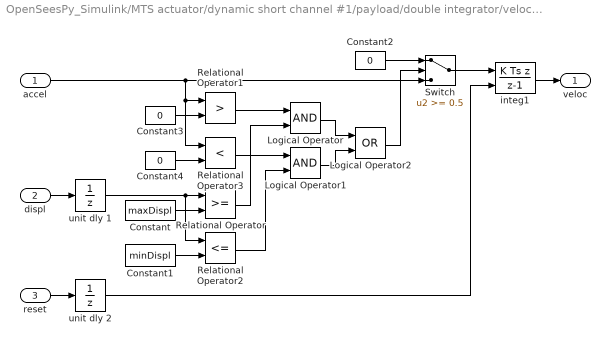
== system OpenSeesPy_Simulink/MTS actuator/dynamic short channel #1/payload/double integrator/veloc gen ==
  accel : Inport
  displ : Inport  Port=2
  reset : Inport  Port=3
  Constant : Constant  Value=maxDispl
  Constant1 : Constant  Value=minDispl
  Constant2 : Constant  Value=0
  Constant3 : Constant  Value=0
  Constant4 : Constant  Value=0
  Logical Operator : Logic
  Logical Operator1 : Logic
  Logical Operator2 : Logic  Operator=OR
  Relational Operator : RelationalOperator  RndMeth=Nearest  InputSameDT=on
  Relational Operator1 : RelationalOperator  Operator=>  RndMeth=Nearest  InputSameDT=on
  Relational Operator2 : RelationalOperator  Operator=<=  RndMeth=Nearest  InputSameDT=on
  Relational Operator3 : RelationalOperator  Operator=<  RndMeth=Nearest  InputSameDT=on
  Switch : Switch  Threshold=0.5  SaturateOnIntegerOverflow=on  InputSameDT=on
  integ1 : DiscreteIntegrator  IntegratorMethod=Integration: Backward Euler  ExternalReset=either  SampleTime=1/1024  LimitOutput=on  UpperSaturationLimit=maxVeloc  LowerSaturationLimit=minVeloc  ICPrevOutput=DiscIntNeverNeededParam  ICPrevScaledInput=DiscIntNeverNeededParam
  unit dly 1 : UnitDelay  SampleTime=-1  HasFrameUpgradeWarning=on
  unit dly 2 : UnitDelay  SampleTime=-1  HasFrameUpgradeWarning=on
  veloc : Outport
  wires:
  integ1/1 -> veloc/1
  Constant/1 -> Relational Operator/2
  Relational Operator/1 -> Logical Operator/2
  Relational Operator2/1 -> Logical Operator1/2
  Constant1/1 -> Relational Operator2/2
  accel/1 -> Relational Operator3/1, Relational Operator1/1, Switch/3
  Constant3/1 -> Relational Operator1/2
  Relational Operator1/1 -> Logical Operator/1
  Constant4/1 -> Relational Operator3/2
  Relational Operator3/1 -> Logical Operator1/1
  Logical Operator/1 -> Logical Operator2/1
  Constant2/1 -> Switch/1
  Logical Operator2/1 -> Switch/2
  Switch/1 -> integ1/1
  unit dly 2/1 -> integ1/2
  Logical Operator1/1 -> Logical Operator2/2
  displ/1 -> unit dly 1/1
  reset/1 -> unit dly 2/1
  unit dly 1/1 -> Relational Operator/1, Relational Operator2/1

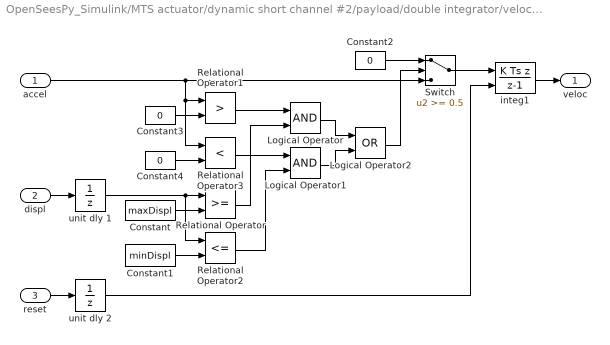
== system OpenSeesPy_Simulink/MTS actuator/dynamic short channel #2/payload/double integrator/veloc gen ==
  accel : Inport
  displ : Inport  Port=2
  reset : Inport  Port=3
  Constant : Constant  Value=maxDispl
  Constant1 : Constant  Value=minDispl
  Constant2 : Constant  Value=0
  Constant3 : Constant  Value=0
  Constant4 : Constant  Value=0
  Logical Operator : Logic
  Logical Operator1 : Logic
  Logical Operator2 : Logic  Operator=OR
  Relational Operator : RelationalOperator  RndMeth=Nearest  InputSameDT=on
  Relational Operator1 : RelationalOperator  Operator=>  RndMeth=Nearest  InputSameDT=on
  Relational Operator2 : RelationalOperator  Operator=<=  RndMeth=Nearest  InputSameDT=on
  Relational Operator3 : RelationalOperator  Operator=<  RndMeth=Nearest  InputSameDT=on
  Switch : Switch  Threshold=0.5  SaturateOnIntegerOverflow=on  InputSameDT=on
  integ1 : DiscreteIntegrator  IntegratorMethod=Integration: Backward Euler  ExternalReset=either  SampleTime=-1  LimitOutput=on  UpperSaturationLimit=maxVeloc  LowerSaturationLimit=minVeloc  ICPrevOutput=DiscIntNeverNeededParam  ICPrevScaledInput=DiscIntNeverNeededParam
  unit dly 1 : UnitDelay  SampleTime=-1  HasFrameUpgradeWarning=on
  unit dly 2 : UnitDelay  SampleTime=-1  HasFrameUpgradeWarning=on
  veloc : Outport
  wires:
  integ1/1 -> veloc/1
  Constant/1 -> Relational Operator/2
  Relational Operator/1 -> Logical Operator/2
  Relational Operator2/1 -> Logical Operator1/2
  Constant1/1 -> Relational Operator2/2
  accel/1 -> Relational Operator3/1, Relational Operator1/1, Switch/3
  Constant3/1 -> Relational Operator1/2
  Relational Operator1/1 -> Logical Operator/1
  Constant4/1 -> Relational Operator3/2
  Relational Operator3/1 -> Logical Operator1/1
  Logical Operator/1 -> Logical Operator2/1
  Constant2/1 -> Switch/1
  Logical Operator2/1 -> Switch/2
  Switch/1 -> integ1/1
  unit dly 2/1 -> integ1/2
  Logical Operator1/1 -> Logical Operator2/2
  displ/1 -> unit dly 1/1
  reset/1 -> unit dly 2/1
  unit dly 1/1 -> Relational Operator/1, Relational Operator2/1

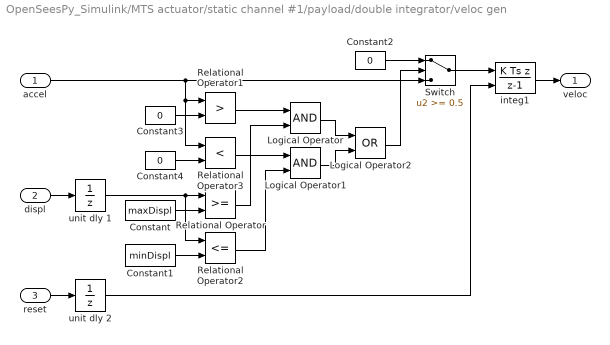
== system OpenSeesPy_Simulink/MTS actuator/static channel #1/payload/double integrator/veloc gen ==
  accel : Inport
  displ : Inport  Port=2
  reset : Inport  Port=3
  Constant : Constant  Value=maxDispl
  Constant1 : Constant  Value=minDispl
  Constant2 : Constant  Value=0
  Constant3 : Constant  Value=0
  Constant4 : Constant  Value=0
  Logical Operator : Logic
  Logical Operator1 : Logic
  Logical Operator2 : Logic  Operator=OR
  Relational Operator : RelationalOperator  RndMeth=Nearest  InputSameDT=on
  Relational Operator1 : RelationalOperator  Operator=>  RndMeth=Nearest  InputSameDT=on
  Relational Operator2 : RelationalOperator  Operator=<=  RndMeth=Nearest  InputSameDT=on
  Relational Operator3 : RelationalOperator  Operator=<  RndMeth=Nearest  InputSameDT=on
  Switch : Switch  Threshold=0.5  SaturateOnIntegerOverflow=on  InputSameDT=on
  integ1 : DiscreteIntegrator  IntegratorMethod=Integration: Backward Euler  ExternalReset=either  SampleTime=-1  LimitOutput=on  UpperSaturationLimit=maxVeloc  LowerSaturationLimit=minVeloc  ICPrevOutput=DiscIntNeverNeededParam  ICPrevScaledInput=DiscIntNeverNeededParam
  unit dly 1 : UnitDelay  SampleTime=-1  HasFrameUpgradeWarning=on
  unit dly 2 : UnitDelay  SampleTime=-1  HasFrameUpgradeWarning=on
  veloc : Outport
  wires:
  integ1/1 -> veloc/1
  Constant/1 -> Relational Operator/2
  Relational Operator/1 -> Logical Operator/2
  Relational Operator2/1 -> Logical Operator1/2
  Constant1/1 -> Relational Operator2/2
  accel/1 -> Relational Operator3/1, Relational Operator1/1, Switch/3
  Constant3/1 -> Relational Operator1/2
  Relational Operator1/1 -> Logical Operator/1
  Constant4/1 -> Relational Operator3/2
  Relational Operator3/1 -> Logical Operator1/1
  Logical Operator/1 -> Logical Operator2/1
  Constant2/1 -> Switch/1
  Logical Operator2/1 -> Switch/2
  Switch/1 -> integ1/1
  unit dly 2/1 -> integ1/2
  Logical Operator1/1 -> Logical Operator2/2
  displ/1 -> unit dly 1/1
  reset/1 -> unit dly 2/1
  unit dly 1/1 -> Relational Operator/1, Relational Operator2/1

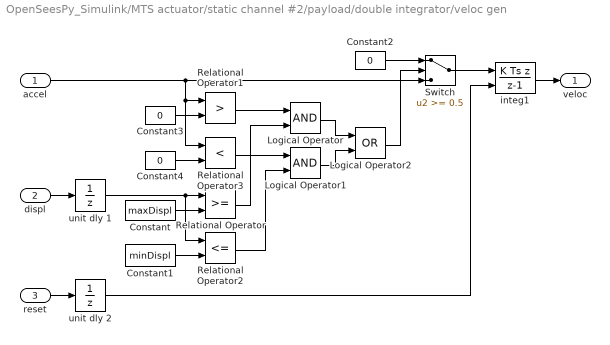
== system OpenSeesPy_Simulink/MTS actuator/static channel #2/payload/double integrator/veloc gen ==
  accel : Inport
  displ : Inport  Port=2
  reset : Inport  Port=3
  Constant : Constant  Value=maxDispl
  Constant1 : Constant  Value=minDispl
  Constant2 : Constant  Value=0
  Constant3 : Constant  Value=0
  Constant4 : Constant  Value=0
  Logical Operator : Logic
  Logical Operator1 : Logic
  Logical Operator2 : Logic  Operator=OR
  Relational Operator : RelationalOperator  RndMeth=Nearest  InputSameDT=on
  Relational Operator1 : RelationalOperator  Operator=>  RndMeth=Nearest  InputSameDT=on
  Relational Operator2 : RelationalOperator  Operator=<=  RndMeth=Nearest  InputSameDT=on
  Relational Operator3 : RelationalOperator  Operator=<  RndMeth=Nearest  InputSameDT=on
  Switch : Switch  Threshold=0.5  SaturateOnIntegerOverflow=on  InputSameDT=on
  integ1 : DiscreteIntegrator  IntegratorMethod=Integration: Backward Euler  ExternalReset=either  SampleTime=-1  LimitOutput=on  UpperSaturationLimit=maxVeloc  LowerSaturationLimit=minVeloc  ICPrevOutput=DiscIntNeverNeededParam  ICPrevScaledInput=DiscIntNeverNeededParam
  unit dly 1 : UnitDelay  SampleTime=-1  HasFrameUpgradeWarning=on
  unit dly 2 : UnitDelay  SampleTime=-1  HasFrameUpgradeWarning=on
  veloc : Outport
  wires:
  integ1/1 -> veloc/1
  Constant/1 -> Relational Operator/2
  Relational Operator/1 -> Logical Operator/2
  Relational Operator2/1 -> Logical Operator1/2
  Constant1/1 -> Relational Operator2/2
  accel/1 -> Relational Operator3/1, Relational Operator1/1, Switch/3
  Constant3/1 -> Relational Operator1/2
  Relational Operator1/1 -> Logical Operator/1
  Constant4/1 -> Relational Operator3/2
  Relational Operator3/1 -> Logical Operator1/1
  Logical Operator/1 -> Logical Operator2/1
  Constant2/1 -> Switch/1
  Logical Operator2/1 -> Switch/2
  Switch/1 -> integ1/1
  unit dly 2/1 -> integ1/2
  Logical Operator1/1 -> Logical Operator2/2
  displ/1 -> unit dly 1/1
  reset/1 -> unit dly 2/1
  unit dly 1/1 -> Relational Operator/1, Relational Operator2/1

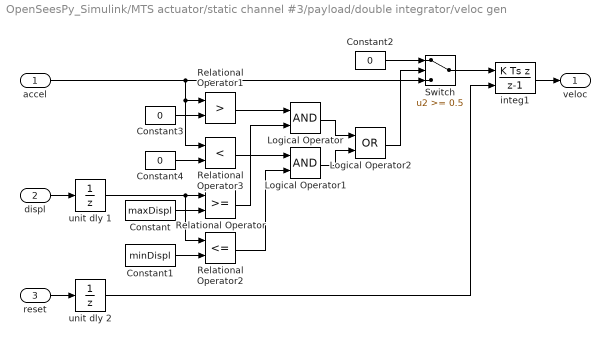
== system OpenSeesPy_Simulink/MTS actuator/static channel #3/payload/double integrator/veloc gen ==
  accel : Inport
  displ : Inport  Port=2
  reset : Inport  Port=3
  Constant : Constant  Value=maxDispl
  Constant1 : Constant  Value=minDispl
  Constant2 : Constant  Value=0
  Constant3 : Constant  Value=0
  Constant4 : Constant  Value=0
  Logical Operator : Logic
  Logical Operator1 : Logic
  Logical Operator2 : Logic  Operator=OR
  Relational Operator : RelationalOperator  RndMeth=Nearest  InputSameDT=on
  Relational Operator1 : RelationalOperator  Operator=>  RndMeth=Nearest  InputSameDT=on
  Relational Operator2 : RelationalOperator  Operator=<=  RndMeth=Nearest  InputSameDT=on
  Relational Operator3 : RelationalOperator  Operator=<  RndMeth=Nearest  InputSameDT=on
  Switch : Switch  Threshold=0.5  SaturateOnIntegerOverflow=on  InputSameDT=on
  integ1 : DiscreteIntegrator  IntegratorMethod=Integration: Backward Euler  ExternalReset=either  SampleTime=-1  LimitOutput=on  UpperSaturationLimit=maxVeloc  LowerSaturationLimit=minVeloc  ICPrevOutput=DiscIntNeverNeededParam  ICPrevScaledInput=DiscIntNeverNeededParam
  unit dly 1 : UnitDelay  SampleTime=-1  HasFrameUpgradeWarning=on
  unit dly 2 : UnitDelay  SampleTime=-1  HasFrameUpgradeWarning=on
  veloc : Outport
  wires:
  integ1/1 -> veloc/1
  Constant/1 -> Relational Operator/2
  Relational Operator/1 -> Logical Operator/2
  Relational Operator2/1 -> Logical Operator1/2
  Constant1/1 -> Relational Operator2/2
  accel/1 -> Relational Operator3/1, Relational Operator1/1, Switch/3
  Constant3/1 -> Relational Operator1/2
  Relational Operator1/1 -> Logical Operator/1
  Constant4/1 -> Relational Operator3/2
  Relational Operator3/1 -> Logical Operator1/1
  Logical Operator/1 -> Logical Operator2/1
  Constant2/1 -> Switch/1
  Logical Operator2/1 -> Switch/2
  Switch/1 -> integ1/1
  unit dly 2/1 -> integ1/2
  Logical Operator1/1 -> Logical Operator2/2
  displ/1 -> unit dly 1/1
  reset/1 -> unit dly 2/1
  unit dly 1/1 -> Relational Operator/1, Relational Operator2/1

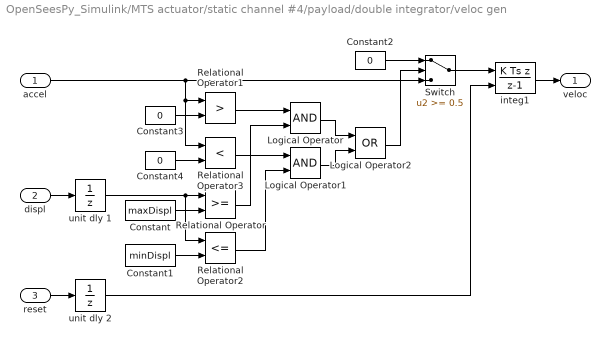
== system OpenSeesPy_Simulink/MTS actuator/static channel #4/payload/double integrator/veloc gen ==
  accel : Inport
  displ : Inport  Port=2
  reset : Inport  Port=3
  Constant : Constant  Value=maxDispl
  Constant1 : Constant  Value=minDispl
  Constant2 : Constant  Value=0
  Constant3 : Constant  Value=0
  Constant4 : Constant  Value=0
  Logical Operator : Logic
  Logical Operator1 : Logic
  Logical Operator2 : Logic  Operator=OR
  Relational Operator : RelationalOperator  RndMeth=Nearest  InputSameDT=on
  Relational Operator1 : RelationalOperator  Operator=>  RndMeth=Nearest  InputSameDT=on
  Relational Operator2 : RelationalOperator  Operator=<=  RndMeth=Nearest  InputSameDT=on
  Relational Operator3 : RelationalOperator  Operator=<  RndMeth=Nearest  InputSameDT=on
  Switch : Switch  Threshold=0.5  SaturateOnIntegerOverflow=on  InputSameDT=on
  integ1 : DiscreteIntegrator  IntegratorMethod=Integration: Backward Euler  ExternalReset=either  SampleTime=-1  LimitOutput=on  UpperSaturationLimit=maxVeloc  LowerSaturationLimit=minVeloc  ICPrevOutput=DiscIntNeverNeededParam  ICPrevScaledInput=DiscIntNeverNeededParam
  unit dly 1 : UnitDelay  SampleTime=-1  HasFrameUpgradeWarning=on
  unit dly 2 : UnitDelay  SampleTime=-1  HasFrameUpgradeWarning=on
  veloc : Outport
  wires:
  integ1/1 -> veloc/1
  Constant/1 -> Relational Operator/2
  Relational Operator/1 -> Logical Operator/2
  Relational Operator2/1 -> Logical Operator1/2
  Constant1/1 -> Relational Operator2/2
  accel/1 -> Relational Operator3/1, Relational Operator1/1, Switch/3
  Constant3/1 -> Relational Operator1/2
  Relational Operator1/1 -> Logical Operator/1
  Constant4/1 -> Relational Operator3/2
  Relational Operator3/1 -> Logical Operator1/1
  Logical Operator/1 -> Logical Operator2/1
  Constant2/1 -> Switch/1
  Logical Operator2/1 -> Switch/2
  Switch/1 -> integ1/1
  unit dly 2/1 -> integ1/2
  Logical Operator1/1 -> Logical Operator2/2
  displ/1 -> unit dly 1/1
  reset/1 -> unit dly 2/1
  unit dly 1/1 -> Relational Operator/1, Relational Operator2/1
